simulink model "SLWINP"  (R2022b)
settings: configuration reference "SharedConfig" (kept outside this file)
values from neighbouring files (symbols this model uses):
  AuxPwrAcvDebFall_C = 0.0    [SLWINP.sldd]
  AuxPwrAcvDebRisng_C = 0.0    [SLWINP.sldd]
  AuxPwrAcvDialEna_C = 1.0    [SLWINP.sldd]
  AuxPwrAcvDialVal_C = 0.0    [SLWINP.sldd]
  AuxPwrStsIvt_C = 0.0    [SLWINP.sldd]
  BdT1DialEna_C = 1.0    [SLWINP.sldd]
  BdT1DialVal_C = 0.0    [SLWINP.sldd]
  BdT1FilTiCon_C = 0.0    [SLWINP.sldd]
  BdT1Gain_C = 1.0    [SLWINP.sldd]
  BdT1Ofs_C = 0.0    [SLWINP.sldd]
  BdT2DialEna_C = 1.0    [SLWINP.sldd]
  BdT2DialVal_C = 0.0    [SLWINP.sldd]
  BdT2FilTiCon_C = 0.0    [SLWINP.sldd]
  BdT2Gain_C = 1.0    [SLWINP.sldd]
  BdT2Ofs_C = 0.0    [SLWINP.sldd]
  DT_SLWINP_C = 0.1    [SLWINP.sldd]
  MaiPwrAcvDebFall_C = 0.0    [SLWINP.sldd]
  MaiPwrAcvDebRisng_C = 0.0    [SLWINP.sldd]
  MaiPwrAcvDialEna_C = 1.0    [SLWINP.sldd]
  MaiPwrAcvDialVal_C = 0.0    [SLWINP.sldd]
  MaiPwrStsIvt_C = 0.0    [SLWINP.sldd]
  McuTDialEna_C = 1.0    [SLWINP.sldd]
  McuTDialVal_C = 0.0    [SLWINP.sldd]
  McuTFilTiCon_C = 0.0    [SLWINP.sldd]
  McuTGain_C = 0.0    [SLWINP.sldd]
  McuTOfs_C = 0.0    [SLWINP.sldd]
  McuUBatFilTiCon_C = 0.0    [SLWINP.sldd]
  McuUBatGain_C = 0.01173    [SLWINP.sldd]
  McuUBatOfs_C = 0.0    [SLWINP.sldd]
  McuURefFilTiCon_C = 0.0    [SLWINP.sldd]
  McuURefGain_C = 0.0    [SLWINP.sldd]
  McuURefOfs_C = 0.0    [SLWINP.sldd]
undefined symbols (not defined in the file or in its folder): slcm
libraries: BlockLibrary x7
Description:
  | Converts raw inputs for the slow rate task into engineering units.
settings Model: DataDictionary=SLWINP.sldd  Creator=Kevin  LastModifiedBy=Max Kolesnikov
settings ConfigSetRef: SourceName=SharedConfig

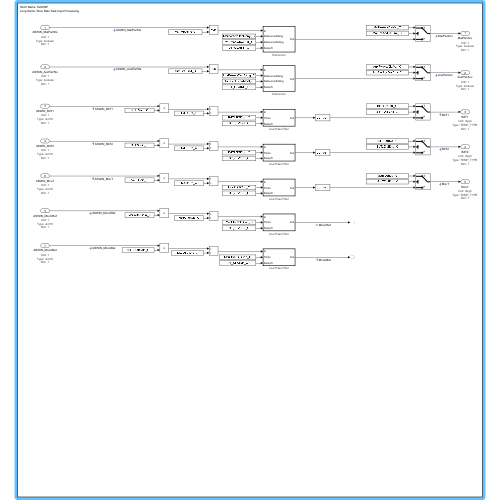
[thumbnail: Simulink's stored preview of the top-level diagram]
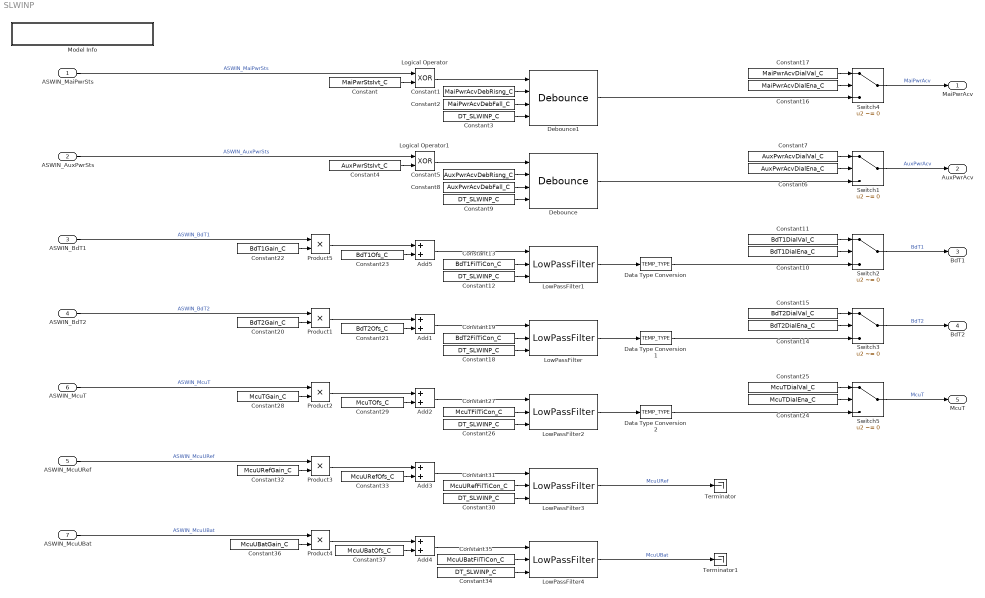
== system SLWINP ==
  ASWIN_MaiPwrSts : Inport  OutDataTypeStr=boolean  Unit=1  PortDimensions=1
      settings: AttributesFormatString=|
      | Unit: %<Unit>
      | Type: %<OutDataTypeStr>
      | Dim: %<PortDimensions>
  ASWIN_AuxPwrSts : Inport  Port=2  OutDataTypeStr=boolean  Unit=1  PortDimensions=1
      settings: AttributesFormatString=|
      | Unit: %<Unit>
      | Type: %<OutDataTypeStr>
      | Dim: %<PortDimensions>
  ASWIN_BdT1 : Inport  Port=3  OutDataTypeStr=uint16  Unit=1  PortDimensions=1
      settings: AttributesFormatString=|
      | Unit: %<Unit>
      | Type: %<OutDataTypeStr>
      | Dim: %<PortDimensions>
  ASWIN_BdT2 : Inport  Port=4  OutDataTypeStr=uint16  Unit=1  PortDimensions=1
      settings: AttributesFormatString=|
      | Unit: %<Unit>
      | Type: %<OutDataTypeStr>
      | Dim: %<PortDimensions>
  ASWIN_McuURef : Inport  Port=5  OutDataTypeStr=uint16  Unit=1  PortDimensions=1
      settings: AttributesFormatString=|
      | Unit: %<Unit>
      | Type: %<OutDataTypeStr>
      | Dim: %<PortDimensions>
  ASWIN_McuT : Inport  Port=6  OutDataTypeStr=uint16  Unit=1  PortDimensions=1
      settings: AttributesFormatString=|
      | Unit: %<Unit>
      | Type: %<OutDataTypeStr>
      | Dim: %<PortDimensions>
  ASWIN_McuUBat : Inport  Port=7  OutDataTypeStr=uint16  Unit=1  PortDimensions=1
      settings: AttributesFormatString=|
      | Unit: %<Unit>
      | Type: %<OutDataTypeStr>
      | Dim: %<PortDimensions>
  Add{1..5} (5 alike) : Sum
  Constant : Constant  Value=MaiPwrStsIvt_C
  Constant1 : Constant  Value=MaiPwrAcvDebRisng_C
  Constant10 : Constant  Value=BdT1DialEna_C
  Constant11 : Constant  Value=BdT1DialVal_C
  Constant{3,9,12,18,26,30,34} (7 alike) : Constant  Value=DT_SLWINP_C
  Constant13 : Constant  Value=BdT1FilTiCon_C
  Constant14 : Constant  Value=BdT2DialEna_C
  Constant15 : Constant  Value=BdT2DialVal_C
  Constant16 : Constant  Value=MaiPwrAcvDialEna_C
  Constant17 : Constant  Value=MaiPwrAcvDialVal_C
  Constant19 : Constant  Value=BdT2FilTiCon_C
  Constant2 : Constant  Value=MaiPwrAcvDebFall_C
  Constant20 : Constant  Value=BdT2Gain_C
  Constant21 : Constant  Value=BdT2Ofs_C
  Constant22 : Constant  Value=BdT1Gain_C
  Constant23 : Constant  Value=BdT1Ofs_C
  Constant24 : Constant  Value=McuTDialEna_C
  Constant25 : Constant  Value=McuTDialVal_C
  Constant27 : Constant  Value=McuTFilTiCon_C
  Constant28 : Constant  Value=McuTGain_C
  Constant29 : Constant  Value=McuTOfs_C
  Constant31 : Constant  Value=McuURefFilTiCon_C
  Constant32 : Constant  Value=McuURefGain_C
  Constant33 : Constant  Value=McuURefOfs_C
  Constant35 : Constant  Value=McuUBatFilTiCon_C
  Constant36 : Constant  Value=McuUBatGain_C
  Constant37 : Constant  Value=McuUBatOfs_C
  Constant4 : Constant  Value=AuxPwrStsIvt_C
  Constant5 : Constant  Value=AuxPwrAcvDebRisng_C
  Constant6 : Constant  Value=AuxPwrAcvDialEna_C
  Constant7 : Constant  Value=AuxPwrAcvDialVal_C
  Constant8 : Constant  Value=AuxPwrAcvDebFall_C
  Data Type Conversion : DataTypeConversion  OutDataTypeStr=TEMP_TYPE  SaturateOnIntegerOverflow=off  RndMeth=Floor
  Data Type Conversion1 : DataTypeConversion  OutDataTypeStr=TEMP_TYPE  SaturateOnIntegerOverflow=off  RndMeth=Floor
  Data Type Conversion2 : DataTypeConversion  OutDataTypeStr=TEMP_TYPE  SaturateOnIntegerOverflow=off  RndMeth=Floor
  Debounce : BlockLibrary/Debounce  Description=Debounce  SystemSampleTime=-1  VariantActivationTime=update diagram  Latency=0  AutoFrameSizeCalculation=off
      settings: AttributesFormatString=%<Description>
  Debounce1 : BlockLibrary/Debounce  Description=Debounce  SystemSampleTime=-1  VariantActivationTime=update diagram  Latency=0  AutoFrameSizeCalculation=off
      settings: AttributesFormatString=%<Description>
  Logical Operator : Logic  Operator=XOR  AllPortsSameDT=off  OutDataTypeStr=boolean
  Logical Operator1 : Logic  Operator=XOR  AllPortsSameDT=off  OutDataTypeStr=boolean
  LowPassFilter{,1..4} (5 alike) : BlockLibrary/LowPassFilter  Description=Low-Pass Filter  SystemSampleTime=-1  VariantActivationTime=update diagram  Latency=0  AutoFrameSizeCalculation=off
      settings: AttributesFormatString=%<Description>
  Model Info : Subsystem  LoadFcn=slcm LoadBlock;  InitFcn=slcm('UpdateAllCMBlocksInThisModelInit')  mask(CMBlock){Frame=off, DisplayStringWithTags=|, MaskDisplayString=Short Name: SLWINP\nLong Name: Slow Rate Task Input Processing, HorizontalTextAlignment=Left, LeftAlignmentValue=0.02}
      mask DisplayStringWithTags=|
      | Short Name: %<ModelName>
      | Long Name: Slow Rate Task Input Processing
      mask prompts: Frame "Simulink:masks:Frame_MP"; DisplayStringWithTags "Simulink:masks:DisplayStringWithTags_MP"; MaskDisplayString "Simulink:masks:MaskDisplayString_MP"; HorizontalTextAlignment "Simulink:masks:HorizontalTextAlignment_MP"; LeftAlignmentValue "Simulink:masks:LeftAlignmentValue_MP"
      mask help: Simulink:masks:CMBlock_MD
      settings: CopyFcn=slcm CopyBlock;  DeleteFcn=slcm Cancel;  PostSaveFcn=slcm('UpdateAllCMBlocksInThisModel')  NameChangeFcn=slcm Rename;  OpenFcn=slcm
      mask Display: text(slResolve(LeftAlignmentValue, gcbh), 0.5, MaskDisplayString, 'HorizontalAlignment', HorizontalTextAlignment)
  Product{1..5} (5 alike) : Product
  Switch{1..5} (5 alike) : Switch  Criteria=u2 ~= 0  SaturateOnIntegerOverflow=off  InputSameDT=off
  Terminator : Terminator
  Terminator1 : Terminator
  MaiPwrAcv : Outport  OutDataTypeStr=boolean  Unit=1  PortDimensions=1
      settings: AttributesFormatString=|
      | Unit: %<Unit>
      | Type: %<OutDataTypeStr>
      | Dim: %<PortDimensions>
  AuxPwrAcv : Outport  Port=2  OutDataTypeStr=boolean  Unit=1  PortDimensions=1
      settings: AttributesFormatString=|
      | Unit: %<Unit>
      | Type: %<OutDataTypeStr>
      | Dim: %<PortDimensions>
  BdT1 : Outport  Port=3  OutDataTypeStr=TEMP_TYPE  Unit=degC  PortDimensions=1
      settings: AttributesFormatString=|
      | Unit: %<Unit>
      | Type: %<OutDataTypeStr>
      | Dim: %<PortDimensions>
  BdT2 : Outport  Port=4  OutDataTypeStr=TEMP_TYPE  Unit=degC  PortDimensions=1
      settings: AttributesFormatString=|
      | Unit: %<Unit>
      | Type: %<OutDataTypeStr>
      | Dim: %<PortDimensions>
  McuT : Outport  Port=5  OutDataTypeStr=TEMP_TYPE  Unit=degC  PortDimensions=1
      settings: AttributesFormatString=|
      | Unit: %<Unit>
      | Type: %<OutDataTypeStr>
      | Dim: %<PortDimensions>
  wires:
  ASWIN_MaiPwrSts/1 -> Logical Operator/1  "ASWIN_MaiPwrSts"
  Constant/1 -> Logical Operator/2
  Logical Operator/1 -> Debounce1/1
  Constant1/1 -> Debounce1/2
  Constant2/1 -> Debounce1/3
  Constant3/1 -> Debounce1/4
  Constant16/1 -> Switch4/2
  Constant17/1 -> Switch4/1
  Debounce1/1 -> Switch4/3
  Switch4/1 -> MaiPwrAcv/1  "MaiPwrAcv"
  Debounce/1 -> Switch1/3
  Constant7/1 -> Switch1/1
  Constant6/1 -> Switch1/2
  Constant9/1 -> Debounce/4
  Constant8/1 -> Debounce/3
  Constant5/1 -> Debounce/2
  Logical Operator1/1 -> Debounce/1
  Constant4/1 -> Logical Operator1/2
  ASWIN_AuxPwrSts/1 -> Logical Operator1/1  "ASWIN_AuxPwrSts"
  Switch1/1 -> AuxPwrAcv/1  "AuxPwrAcv"
  Product5/1 -> Add5/1
  Constant23/1 -> Add5/2
  Constant22/1 -> Product5/2
  ASWIN_BdT1/1 -> Product5/1  "ASWIN_BdT1"
  Add5/1 -> LowPassFilter1/1
  Constant10/1 -> Switch2/2
  Constant11/1 -> Switch2/1
  LowPassFilter1/1 -> Data Type Conversion/1
  Constant12/1 -> LowPassFilter1/3
  Constant13/1 -> LowPassFilter1/2
  Switch2/1 -> BdT1/1  "BdT1"
  Switch3/1 -> BdT2/1  "BdT2"
  Constant19/1 -> LowPassFilter/2
  Constant18/1 -> LowPassFilter/3
  LowPassFilter/1 -> Data Type Conversion1/1
  Constant15/1 -> Switch3/1
  Constant14/1 -> Switch3/2
  Add1/1 -> LowPassFilter/1
  ASWIN_BdT2/1 -> Product1/1  "ASWIN_BdT2"
  Constant20/1 -> Product1/2
  Constant21/1 -> Add1/2
  Product1/1 -> Add1/1
  Product2/1 -> Add2/1
  Constant29/1 -> Add2/2
  Constant28/1 -> Product2/2
  ASWIN_McuT/1 -> Product2/1  "ASWIN_McuT"
  Add2/1 -> LowPassFilter2/1
  Constant24/1 -> Switch5/2
  Constant25/1 -> Switch5/1
  LowPassFilter2/1 -> Data Type Conversion2/1
  Constant26/1 -> LowPassFilter2/3
  Constant27/1 -> LowPassFilter2/2
  Switch5/1 -> McuT/1  "McuT"
  Constant31/1 -> LowPassFilter3/2
  Constant30/1 -> LowPassFilter3/3
  Add3/1 -> LowPassFilter3/1
  ASWIN_McuURef/1 -> Product3/1  "ASWIN_McuURef"
  Constant32/1 -> Product3/2
  Constant33/1 -> Add3/2
  Product3/1 -> Add3/1
  Product4/1 -> Add4/1
  Constant37/1 -> Add4/2
  Constant36/1 -> Product4/2
  ASWIN_McuUBat/1 -> Product4/1  "ASWIN_McuUBat"
  Add4/1 -> LowPassFilter4/1
  Constant34/1 -> LowPassFilter4/3
  Constant35/1 -> LowPassFilter4/2
  Data Type Conversion/1 -> Switch2/3
  Data Type Conversion1/1 -> Switch3/3
  Data Type Conversion2/1 -> Switch5/3
  LowPassFilter3/1 -> Terminator/1  "McuURef"
  LowPassFilter4/1 -> Terminator1/1  "McuUBat"

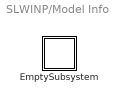
== system SLWINP/Model Info ==
  EmptySubsystem : Subsystem

== system SLWINP/Model Info/EmptySubsystem ==
